simulink library "libConditions"  (R2013a)
settings: Solver=ode45  StartTime=0.0  StopTime=10.0  RelTol=1e-3
libraries: libUtilities x1
settings Model: Creator=shenoylab  LastModifiedBy=shenoylab

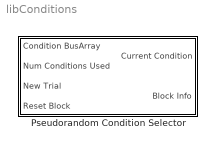
== system libConditions ==
  Pseudorandom Condition Selector : Subsystem

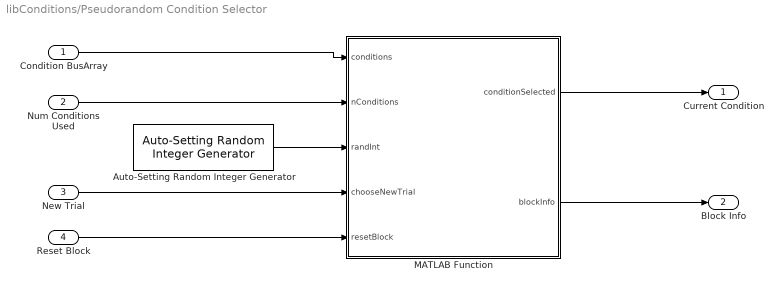
== system libConditions/Pseudorandom Condition Selector ==
  Condition BusArray : Inport  OutDataTypeStr=Bus: ConditionBus
  Num Conditions Used : Inport  Port=2  OutDataTypeStr=uint16  PortDimensions=1
  New Trial : Inport  Port=3  OutDataTypeStr=uint8  PortDimensions=1
  Reset Block : Inport  Port=4  OutDataTypeStr=uint8  PortDimensions=1
  Auto-Setting Random Integer Generator : libUtilities/Auto-Setting Random Integer Generator  mul=2^32  Ts=0.001  outDataType=uint32
  MATLAB Function : MATLAB Function  TreatAsAtomicUnit=on
  Current Condition : Outport
  Block Info : Outport  Port=2
  wires:
  Auto-Setting Random Integer Generator/1 -> MATLAB Function/3(randInt)
  MATLAB Function/1(conditionSelected) -> Current Condition/1
  MATLAB Function/2(blockInfo) -> Block Info/1
  Num Conditions Used/1 -> MATLAB Function/2(nConditions)
  Condition BusArray/1 -> MATLAB Function/1(conditions)
  Reset Block/1 -> MATLAB Function/5(resetBlock)
  New Trial/1 -> MATLAB Function/4(chooseNewTrial)

== matlab function libConditions/Pseudorandom Condition Selector/MATLAB Function ==
  data: conditions input Bus: ConditionBus; nConditions input uint16 size=1; randInt input uint32 size=1; chooseNewTrial input uint8 size=1; conditionSelected output Bus: ConditionBus size=1; blockInfo output Bus: BlockInfoBus; resetBlock input uint8 size=1
function [conditionSelected, blockInfo] = pseudorandomSelect(conditions, nConditions, randInt, chooseNewTrial, resetBlock)
%#codegen

% store original conditions inputs, as well as a copy we can modify locally
persistent pConditionsOriginal;
persistent pNConditionsOriginal;
persistent pConditions;
persistent pNConditions;

persistent pBlockInfo;
persistent pConditionCurrent;

if isempty(pConditionsOriginal) || isempty(pNConditionsOriginal) 
    pConditionsOriginal = conditions;
    pNConditionsOriginal = nConditions;
    pConditions = conditions;
    pNConditions = nConditions;
    chooseNewTrial = uint8(1);
    
elseif ~isequal(pConditionsOriginal, conditions) || pNConditionsOriginal ~= nConditions
    % changes has been made to tunable conditions bus via tuning,
    % reset the blocks
    pConditionsOriginal = conditions;
    pNConditionsOriginal = nConditions;
    pConditions = conditions;
    pNConditions = nConditions;
    chooseNewTrial = uint8(1);
end

if isempty(pBlockInfo)
    pBlockInfo.nTrialsRemaining = uint16(0);
    pBlockInfo.nBlocksCompleted = uint16(0);
end

if isempty(pConditionCurrent)
    pConditionCurrent = uint16(1);
    chooseNewTrial = uint8(1);
end
    
if resetBlock
    pConditions = pConditionsOriginal;
    pNConditions = pNConditions;
end

% compute number of trials remaining in block
pBlockInfo.nTrialsRemaining = uint16(0);
for iC = uint16(1):uint16(pNConditions)
    pBlockInfo.nTrialsRemaining = pBlockInfo.nTrialsRemaining + uint16(pConditions(iC).conditionRepeats);
end

if chooseNewTrial
    % check whether we're starting a new block currently
    if pBlockInfo.nTrialsRemaining == uint16(0)
        pConditions = conditions;
        pBlockInfo.nBlocksCompleted = pBlockInfo.nBlocksCompleted + uint16(1);
        for iC1 = uint16(1):uint16(pNConditions)
            pBlockInfo.nTrialsRemaining = pBlockInfo.nTrialsRemaining + uint16(pConditions(iC1).conditionRepeats);
        end
    end
    
    % use the cumulative trial repetitions count (summing over conditions)
    % to choose a trial from the set of reps still to do
    selectorIdx = uint16(mod(randInt, uint32(pBlockInfo.nTrialsRemaining))) + 1;
    cumulativeReps = uint16(0);
    for iC2 = uint16(1):uint16(pNConditions)
        cumulativeReps = cumulativeReps + uint16(pConditions(iC2).conditionRepeats);
        if cumulativeReps >= selectorIdx
            pConditionCurrent = iC2;
            break;
        end
    end   
    
    % subtract one from the condition repeats bus
    pConditions(pConditionCurrent).conditionRepeats = pConditions(pConditionCurrent).conditionRepeats - ...
        cast(1, class(pConditions(pConditionCurrent).conditionRepeats));
    
    pBlockInfo.nTrialsRemaining = pBlockInfo.nTrialsRemaining - uint16(1);
end

conditionSelected = pConditions(pConditionCurrent);
blockInfo = pBlockInfo;
